simulink model "Motor_pos_str_d"  (R2016a)
settings: Solver=ode5  StartTime=0.0  StopTime=20.0  FixedStep=0.005  RelTol=1e-3
settings Model: Creator=Trong  LastModifiedBy=Trong

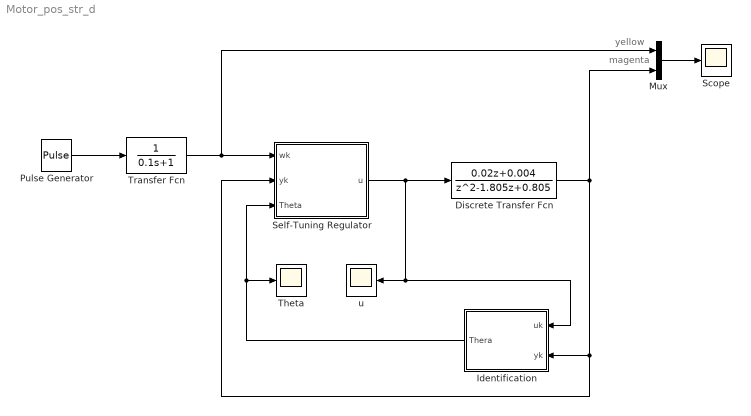
== system Motor_pos_str_d ==
  note: magenta
  note: yellow
  Discrete Transfer Fcn : DiscreteTransferFcn  Numerator=[0.02 0.004]  Denominator=[1 -1.805 0.805]  SampleTime=0.005
  Identification : Subsystem
  Mux : Mux  Inputs=2
  Pulse Generator : DiscretePulseGenerator  PulseType=Time based  Period=4  PulseWidth=50
  Scope : Scope
  Self-Tuning Regulator : Subsystem
  Theta : Scope
  Transfer Fcn : TransferFcn  Denominator=[0.1 1]
  u : Scope
  wires:
  Pulse Generator/1 -> Transfer Fcn/1
  Transfer Fcn/1 -> Mux/1, Self-Tuning Regulator/1(wk)
  Self-Tuning Regulator/1(u) -> u/1, Identification/1(uk), Discrete Transfer Fcn/1
  Discrete Transfer Fcn/1 -> Mux/2, Self-Tuning Regulator/2(yk), Identification/2(yk)
  Mux/1 -> Scope/1
  Identification/1(Thera) -> Self-Tuning Regulator/3(Theta), Theta/1

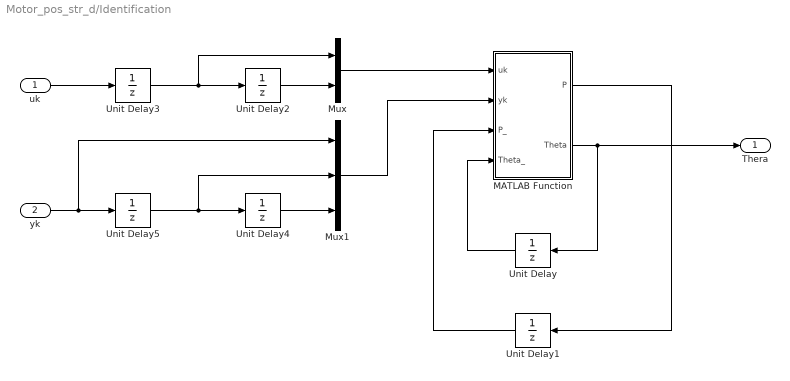
== system Motor_pos_str_d/Identification ==
  uk : Inport
  yk : Inport  Port=2
  MATLAB Function : MATLAB Function  TreatAsAtomicUnit=on
  Mux : Mux  Inputs=2
  Mux1 : Mux  Inputs=3
  Unit Delay : UnitDelay  InitialCondition=rand(4,1)  SampleTime=-1
  Unit Delay1 : UnitDelay  InitialCondition=10^5*eye(4)  SampleTime=-1
  Unit Delay{2..5} (4 alike) : UnitDelay  SampleTime=-1
  Thera : Outport
  wires:
  uk/1 -> Unit Delay3/1
  Unit Delay3/1 -> Mux/1, Unit Delay2/1
  yk/1 -> Mux1/1, Unit Delay5/1
  Unit Delay2/1 -> Mux/2
  Unit Delay5/1 -> Mux1/2, Unit Delay4/1
  MATLAB Function/2(Theta) -> Unit Delay/1, Thera/1
  MATLAB Function/1(P) -> Unit Delay1/1
  Unit Delay/1 -> MATLAB Function/4(Theta_)
  Unit Delay1/1 -> MATLAB Function/3(P_)
  Unit Delay4/1 -> Mux1/3
  Mux/1 -> MATLAB Function/1(uk)
  Mux1/1 -> MATLAB Function/2(yk)

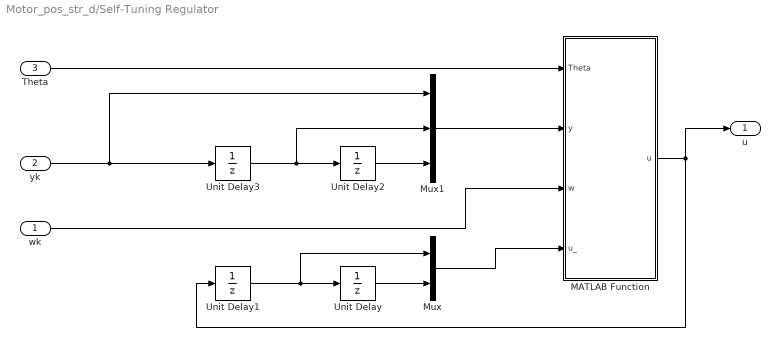
== system Motor_pos_str_d/Self-Tuning Regulator ==
  wk : Inport
  yk : Inport  Port=2
  Theta : Inport  Port=3
  MATLAB Function : MATLAB Function  TreatAsAtomicUnit=on
  Mux : Mux  Inputs=2
  Mux1 : Mux  Inputs=3
  Unit Delay{,1..3} (4 alike) : UnitDelay  SampleTime=-1
  u : Outport
  wires:
  Unit Delay/1 -> Mux/2
  Unit Delay1/1 -> Mux/1, Unit Delay/1
  MATLAB Function/1(u) -> u/1, Unit Delay1/1
  Theta/1 -> MATLAB Function/1(Theta)
  Mux/1 -> MATLAB Function/4(u_)
  Unit Delay2/1 -> Mux1/3
  Unit Delay3/1 -> Mux1/2, Unit Delay2/1
  Mux1/1 -> MATLAB Function/2(y)
  yk/1 -> Mux1/1, Unit Delay3/1
  wk/1 -> MATLAB Function/3(w)

== matlab function Motor_pos_str_d/Self-Tuning Regulator/MATLAB Function ==
  data: Theta input; u output; y input size=3; w input; u_ input size=2
function u = STR_pp1(Theta,y,w,u_)
alpha = 0.7;
beta = 0.7;

% Gan lai thong so de thuan tien viec tinh toan
a1 = Theta(1);
a2 = Theta(2);
b1 = Theta(3);
b2 = Theta(4);

% Tinh thong so bo dieu khien
x1 = -4*alpha+1-a1;
x2 = 6*alpha^2+beta^2+a1-a2;
x3 = 2*alpha*(2*alpha^2+beta^2)-a2;
x4 = alpha^2*(alpha^2+beta^2);
r0 = (x1+x2-x3+x4)/(b1+b2);
r1 = (b1+b2)*(a1*b1*b2-a2*b1^2-b2^2);
r2 = a1*b2*(b1*(x2-x3+x4)-b2*x1);
r3 = a2*b1*(b2*x1-b1*(x2-x3+x4));
r4 = (b1+b2)*(b1*x4+b2*(x3-x4));
r5 = b1*(b1^2*x4+ b1*b2*x3+ b2^2*x2)-b2^3*x1;
r6 = b1^2*(a2*x3+a1*x4-a2*x4);
r7 = b2*(b1*(a1*x4+a2*x2-x4)-b2*(a2*x1+x4));
p1 = (r5-r1)/r1;
p2 = -r5/r1;
q0 = r0-(r2+r3+r4)/r1;
q1 = (r2+r3+r4-r6-r7)/r1;
q2 = (r6+r7)/r1;

% Luat dieu khien
u = r0*w(1) - q0*y(1) - q1*y(2) - q2*y(3) -p1*u_(1) - p2*u_(2);

== matlab function Motor_pos_str_d/Identification/MATLAB Function ==
  data: uk input size=2; P output; yk input size=3; P_ input; Theta_ input; Theta output
% Ham nhan dang thong so doi tuong
function [P,Theta] = Uocluong(uk,yk,P_,Theta_)

lamda = 0.96;

PHI = [-yk(2); -yk(3); uk(1); uk(2)];
e = yk(1) - PHI'*Theta_;
L = P_*PHI / (lamda + PHI'*P_*PHI);
P = 1/lamda*(P_ - P_*PHI*PHI'*P_ /(lamda + PHI'*P_*PHI));
Theta = Theta_ + L*e;
